simulink model "Demodulation_AM"  (R2023a)
settings: Solver=VariableStepAuto  StartTime=0.0  StopTime=1  RelTol=1e-3
libraries: commchan3 x1, dspfdesign x1
settings Model: Creator=dung  LastModifiedBy=dung

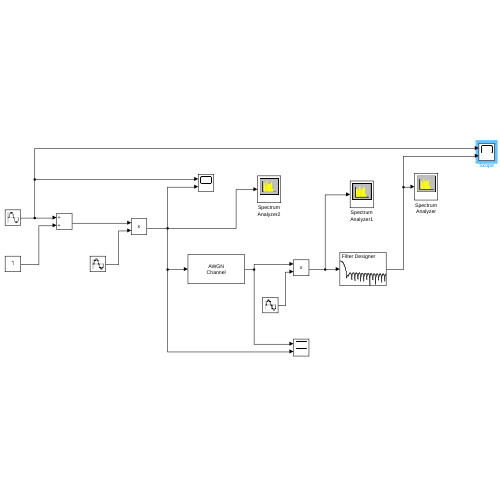
[thumbnail: Simulink's stored preview of the top-level diagram]
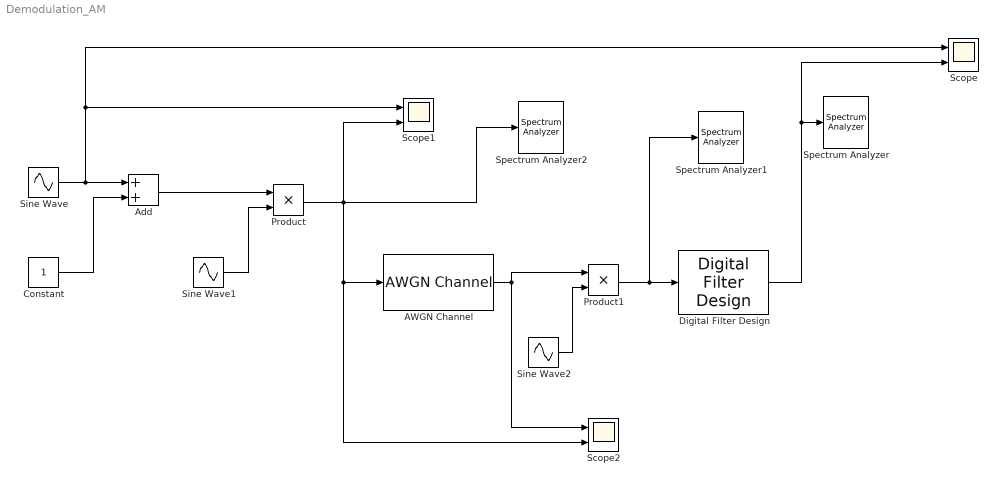
== system Demodulation_AM ==
  AWGN Channel : commchan3/AWGN Channel  LegacyMode=off  NoiseMethod=Variance  noiseMode="Signal to noise ratio  (SNR)"  EbNo=10  EsNo=10  SNR=15  BitsPerSymbol=1  SignalPower=1  SamplesPerSymbol=1  SymbolPeriod=1  VarianceSource=Parameter  Variance=1  RandomStream=mt19937ar with seed  Seed=73  SimulateUsing=Interpreted execution
  Add : Sum
  Constant : Constant
  Digital Filter Design : dspfdesign/Digital Filter Design  mwdsp_browser_bugfix_var=off
  Product : Product
  Product1 : Product
  Scope : Scope  NumInputPorts=2
  Scope1 : Scope  NumInputPorts=2
  Scope2 : Scope  NumInputPorts=2
  Sine Wave : Sin  Frequency=2*pi*200  SampleTime=1/50000
  Sine Wave1 : Sin  Frequency=2*pi*5000  SampleTime=1/50000
  Sine Wave2 : Sin  Frequency=2*pi*5000  SampleTime=1/50000
  Spectrum Analyzer : SpectrumAnalyzer  WindowPosition=[1.000000,1.000000,1863.000000,1016.000000,]  ScopeFrameLocation=window  YLimits=[-96.036576,37.2034049]  ColorLimits=[-20 80]  DefaultConfigurationName=spbscopes.SpectrumAnalyzerBlockCfg  IsFrequencyInputMode=0  FrequencyVectorPort=0  FrequencyVectorFromPort=0  FrequencyInputRBWPort=0  FrequencyInputRBWFromPort=0
  Spectrum Analyzer1 : SpectrumAnalyzer  WindowPosition=[590.000000,215.000000,800.000000,500.000000,]  ScopeFrameLocation=window  YLimits=[-10.03741666,27.78844564]  ColorLimits=[-20 80]  DefaultConfigurationName=spbscopes.SpectrumAnalyzerBlockCfg  IsFrequencyInputMode=0  FrequencyVectorPort=0  FrequencyVectorFromPort=0  FrequencyInputRBWPort=0  FrequencyInputRBWFromPort=0
  Spectrum Analyzer2 : SpectrumAnalyzer  WindowPosition=[129.000000,88.000000,1217.000000,687.000000,]  ScopeFrameLocation=window  YLimits=[-76.85735671,33.23435856]  ColorLimits=[-20 80]  DefaultConfigurationName=spbscopes.SpectrumAnalyzerBlockCfg  IsFrequencyInputMode=0  FrequencyVectorPort=0  FrequencyVectorFromPort=0  FrequencyInputRBWPort=0  FrequencyInputRBWFromPort=0
  wires:
  Sine Wave/1 -> Scope/1, Scope1/1, Add/1
  Constant/1 -> Add/2
  Sine Wave1/1 -> Product/2
  Product/1 -> Spectrum Analyzer2/1, Scope1/2, Scope2/2, AWGN Channel/1
  AWGN Channel/1 -> Product1/1, Scope2/1
  Sine Wave2/1 -> Product1/2
  Product1/1 -> Spectrum Analyzer1/1, Digital Filter Design/1
  Digital Filter Design/1 -> Scope/2, Spectrum Analyzer/1
  Add/1 -> Product/1
